simulink model "lab2ex5"  (R2023b)
settings: Solver=VariableStepAuto  StartTime=0.0  StopTime=65  RelTol=1e-3
settings Model: Creator=shaanyadav  LastModifiedBy=shaanyadav

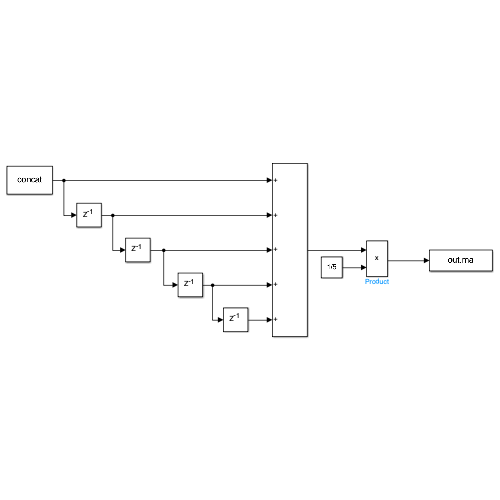
[thumbnail: Simulink's stored preview of the top-level diagram]
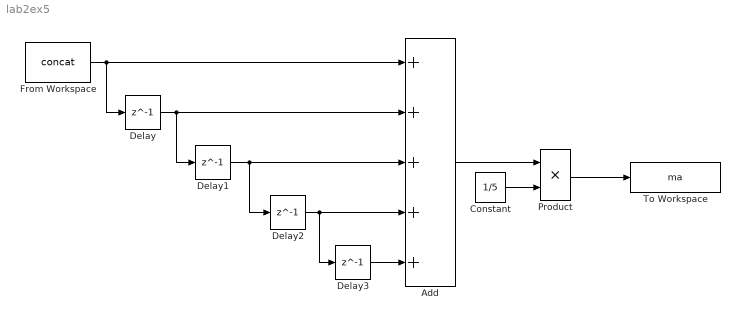
== system lab2ex5 ==
  Add : Sum  Inputs=+++++
  Constant : Constant  Value=1/5
  Delay{,1..3} (4 alike) : Delay  DelayLength=1  InitialCondition=0
  From Workspace : FromWorkspace  VariableName=concat  SampleTime=1
  Product : Product
  To Workspace : ToWorkspace  VariableName=ma  SampleTime=-1
  wires:
  From Workspace/1 -> Delay/1, Add/1
  Delay/1 -> Delay1/1, Add/2
  Delay1/1 -> Delay2/1, Add/3
  Delay2/1 -> Delay3/1, Add/4
  Delay3/1 -> Add/5
  Add/1 -> Product/1
  Product/1 -> To Workspace/1
  Constant/1 -> Product/2
